simulink subsystem "RL_Load_Diff"  (R2021b)
settings: Solver=VariableStepAuto  StartTime=0.0  StopTime=10.0  RelTol=1e-3
undefined symbols (not defined in the file): df, dr, hg, krfr, M, rcf, rch, rcr, WBf
libraries: simulink x2
settings Model: Creator=tsuyoshi  LastModifiedBy=tsuyoshi

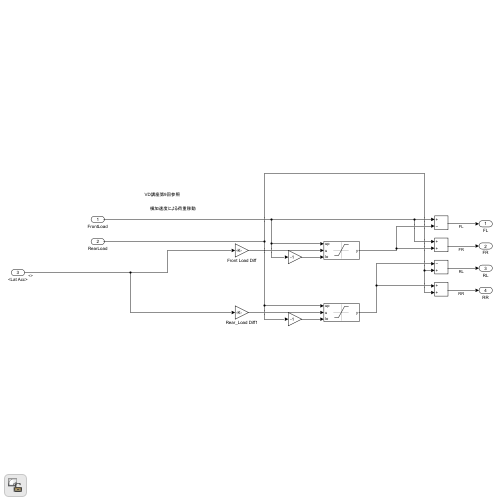
[thumbnail: Simulink's stored preview of the top-level diagram]
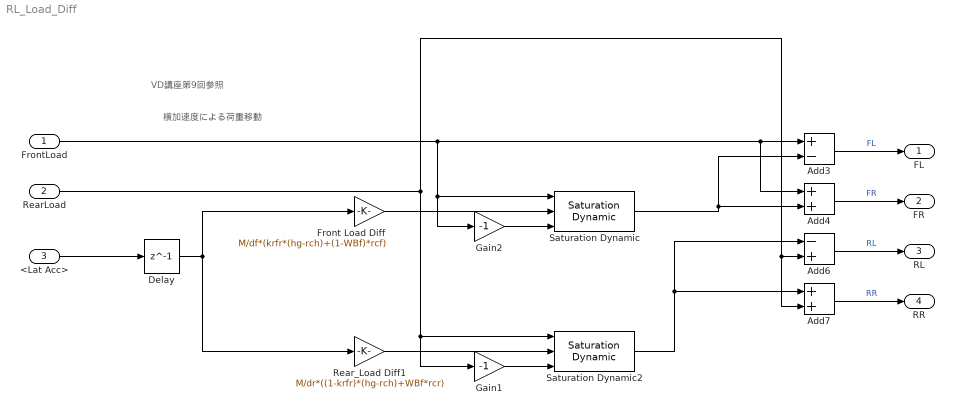
== system RL_Load_Diff ==
  note: 横加速度による荷重移動
  note: VD講座第9回参照
  FrontLoad : Inport
  RearLoad : Inport  Port=2
  <Lat Acc> : Inport  Port=3
  Add3 : Sum  Inputs=+-
  Add4 : Sum
  Add6 : Sum  Inputs=-+
  Add7 : Sum
  Delay : Delay  DelayLength=1
  Front Load Diff : Gain  Gain=M/df*(krfr*(hg-rch)+(1-WBf)*rcf)
  Gain1 : Gain  Gain=-1
  Gain2 : Gain  Gain=-1
  Rear_Load Diff1 : Gain  Gain=M/dr*((1-krfr)*(hg-rch)+WBf*rcr)
  Saturation Dynamic : simulink/Discontinuities/Saturation Dynamic  OutMin=[]  OutMax=[]  OutDataTypeStr=Inherit: Same as second input  OutDataType=fixdt(1, 16)  OutScaling=2^-10  DoSatur=off
  Saturation Dynamic2 : simulink/Discontinuities/Saturation Dynamic  OutMin=[]  OutMax=[]  OutDataTypeStr=Inherit: Same as second input  OutDataType=fixdt(1, 16)  OutScaling=2^-10  DoSatur=off
  FL : Outport
  FR : Outport  Port=2
  RL : Outport  Port=3
  RR : Outport  Port=4
  wires:
  Saturation Dynamic/1 -> Add4/2, Add3/2
  Saturation Dynamic2/1 -> Add7/1, Add6/1
  Rear_Load Diff1/1 -> Saturation Dynamic2/2
  RearLoad/1 -> Add7/2, Add6/2, Gain1/1, Saturation Dynamic2/1
  Front Load Diff/1 -> Saturation Dynamic/2
  FrontLoad/1 -> Add3/1, Add4/1, Gain2/1, Saturation Dynamic/1
  Gain2/1 -> Saturation Dynamic/3
  <Lat Acc>/1 -> Delay/1
  Gain1/1 -> Saturation Dynamic2/3
  Add4/1 -> FR/1  "FR"
  Add6/1 -> RL/1  "RL"
  Add7/1 -> RR/1  "RR"
  Add3/1 -> FL/1  "FL"
  Delay/1 -> Front Load Diff/1, Rear_Load Diff1/1
